simulink model "model_problem8"  (R2020a)
settings: Solver=VariableStepAuto  StartTime=0.0  StopTime=10.0  RelTol=1e-3
settings Model: Creator=Prateek  LastModifiedBy=Prateek

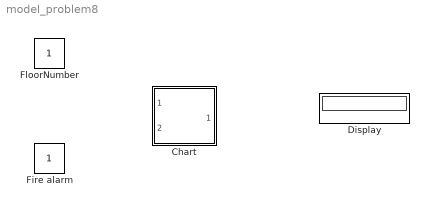
== system model_problem8 ==
  Chart : Stateflow chart  TreatAsAtomicUnit=on
  Display : Display
  Fire alarm : Constant
  FloorNumber : Constant

== stateflow chart model_problem8/Chart ==
  state elevatorON
    state ground_Floor
      entry:
      status=1;
      during:
      presentFloor=0;
      findFloor(presentFloor);
      exit:
      status=0;
    state first_Floor
      entry:
      status=1;
      during:
      presentFloor=1;
      findFloor(presentFloor);
      exit:
      status=0;
    state second_Floor
      entry:
      status=1;
      during:
      presentFloor=2;
      findFloor(presentFloor);
      exit:
      status=0;
    state third_Floor
      entry:
      status=1;
      during:
      presentFloor=3;
      findFloor(presentFloor);
      exit:
      status=0;
    state fourth_Floor
      entry:
      status=1;
      during:
      presentFloor=4;
      findFloor(presentFloor);
      exit:
      status=0;
    state fifth_floor
      entry:
      status=1;
      during:
      presentFloor=5;
      findFloor(presentFloor);
      exit:
      status=0;
    (default) -> ground_Floor
    first_Floor -> ground_Floor [order 2] : down
    ground_Floor -> first_Floor : up
    second_Floor -> first_Floor [order 1] : down
    first_Floor -> second_Floor [order 1] : up
    third_Floor -> second_Floor [order 1] : down
    second_Floor -> third_Floor [order 2] : up
    fourth_Floor -> third_Floor [order 1] : down
    third_Floor -> fourth_Floor [order 2] : up
    fifth_floor -> fourth_Floor : down
    fourth_Floor -> fifth_floor [order 2] : up
  state elevatorOFF
  state Alarm
    (default) -> (junction 55)
    (junction 55) -> (junction 57)
    (junction 57) -> (junction 58)
    (junction 58) -> (junction 59) [order 1] : [alarm==1]{send(off)}
    (junction 58) -> (junction 60) [order 2] : [alarm==0]{send(on)}
    (junction 59) -> (junction 61)
    (junction 61) -> (junction 60)
  state y= findFloor(floor) [function]
    (default) -> (junction 26)
    (junction 26) -> (junction 30) [order 2] : [FloorNumber>floor]{
        | send(up);
        | disp('elevatorUp');}
    (junction 26) -> (junction 29) [order 1] : [FloorNumber<floor]{
        | send(down);
        | disp('elevatorDown');}
    (junction 29) -> (junction 34)
    (junction 26) -> (junction 28) [order 3] : [FloorNumber==floor]{
        | disp('destination');}
    (junction 30) -> (junction 35)
    (junction 34) -> (junction 28)
    (junction 35) -> (junction 28)
    (junction 28) -> (junction 41)
  (default) -> elevatorON
  elevatorON -> elevatorOFF : [FireAlarm==1]
  elevatorOFF -> elevatorON : [FireAlarm==0]
  data: y function_output; floor function_input; findFloor input; status output; presentFloor local; FireAlarm input; alarm local
  events: up local FUNCTION_CALL_EVENT; down local FUNCTION_CALL_EVENT; on local FUNCTION_CALL_EVENT; off local FUNCTION_CALL_EVENT
